simulink model "pendulum"  (R2020b)
settings: Solver=ode45  StartTime=0.0  StopTime=1000  FixedStep=0.01  RelTol=1e-3
InitFcn:
  | init_params
values from neighbouring files (symbols this model uses):
  b = 0.15    [init_params.m]
  g = 9.8    [init_params.m]
  I = 6250000    [init_params.m]
  L = 25    [init_params.m]
  m = 30000    [init_params.m]
  M = 20000    [init_params.m]
libraries: fuzblock x2, simulink_extras x2
settings Model: Creator=Administrator  LastModifiedBy=HZQ
settings SolverCC: ZeroCrossAlgorithm=Adaptive
settings DataIOCC: ReturnWorkspaceOutputs=off
settings DebuggingCC: ArithmeticOperatorsInVariantConditions=warning
settings SFSimCC: CustomCodeUndefinedFunction=UseInterfaceOnly

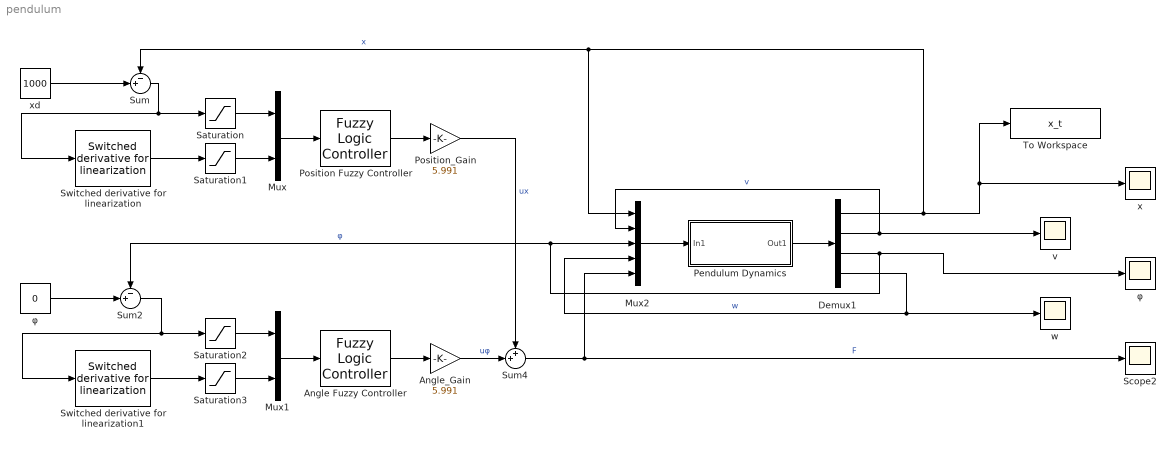
== system pendulum ==
  Angle Fuzzy Controller : fuzblock/Fuzzy Logic  Controller  FIS='angle_fuzzy_trimf.fis'  OutputSampleNumber=101  DataType=double  FuzzifiedInputs=off  RuleFiringStrengths=off  RuleOutputs=off  AggregatedOutputs=off  SimulateUsing=Interpreted execution  OutOfRangeInputValueMessage=warning  NoRuleFiredMessage=warning  EmptyOutputFuzzySetMessage=warning
  Angle_Gain : Gain  Gain=5.991
  Demux1 : Demux
  Mux : Mux  Inputs=2
  Mux1 : Mux  Inputs=2
  Mux2 : Mux  Inputs=5
  Pendulum Dynamics : Subsystem
  Position Fuzzy Controller : fuzblock/Fuzzy Logic  Controller  FIS='position_fuzzy_trimf.fis'  OutputSampleNumber=101  DataType=double  FuzzifiedInputs=off  RuleFiringStrengths=off  RuleOutputs=off  AggregatedOutputs=off  SimulateUsing=Interpreted execution  OutOfRangeInputValueMessage=warning  NoRuleFiredMessage=warning  EmptyOutputFuzzySetMessage=warning
  Position_Gain : Gain  Gain=5.991
  Saturation : Saturate  UpperLimit=1200  LowerLimit=-1200
  Saturation1 : Saturate  UpperLimit=10  LowerLimit=-10
  Saturation2 : Saturate  UpperLimit=6  LowerLimit=-6
  Saturation3 : Saturate  UpperLimit=6  LowerLimit=-6
  Scope2 : Scope
  Sum : Sum  Inputs=-+|
  Sum2 : Sum  Inputs=-+|
  Sum4 : Sum  Inputs=++|
  Switched derivative for linearization : simulink_extras/Linearization/Switched derivative for linearization  switchVal=0  derivConst=100
      settings: SourceProductBaseCode=SL
  Switched derivative for linearization1 : simulink_extras/Linearization/Switched derivative for linearization  switchVal=0  derivConst=100
      settings: SourceProductBaseCode=SL
  To Workspace : ToWorkspace  VariableName=x_t  SaveFormat=Timeseries  SampleTime=-1
  v : Scope
  w : Scope
  x : Scope
  "xd " : Constant  Value=1000  OutDataTypeStr=Inherit: Inherit via back propagation
  φ : Scope
  "φ " : Constant  Value=0  OutDataTypeStr=Inherit: Inherit via back propagation
  wires:
  Mux1/1 -> Angle Fuzzy Controller/1
  Mux/1 -> Position Fuzzy Controller/1
  Pendulum Dynamics/1(Out1) -> Demux1/1
  Demux1/1 -> x/1, To Workspace/1, Sum/1, Mux2/1  "x"
  "xd "/1 -> Sum/2
  Demux1/3 -> Sum2/1, Mux2/3, φ/1  "φ"
  "φ "/1 -> Sum2/2
  Mux2/1 -> Pendulum Dynamics/1(In1)
  Sum4/1 -> Mux2/5, Scope2/1  "F"
  Position Fuzzy Controller/1 -> Position_Gain/1
  Angle Fuzzy Controller/1 -> Angle_Gain/1
  Sum/1 -> Saturation/1, Switched derivative for linearization/1
  Sum2/1 -> Saturation2/1, Switched derivative for linearization1/1
  Position_Gain/1 -> Sum4/1  "ux"
  Angle_Gain/1 -> Sum4/2  "uφ"
  Demux1/2 -> v/1, Mux2/2  "v"
  Demux1/4 -> w/1, Mux2/4  "w"
  Switched derivative for linearization1/1 -> Saturation3/1
  Switched derivative for linearization/1 -> Saturation1/1
  Saturation/1 -> Mux/1
  Saturation1/1 -> Mux/2
  Saturation2/1 -> Mux1/1
  Saturation3/1 -> Mux1/2

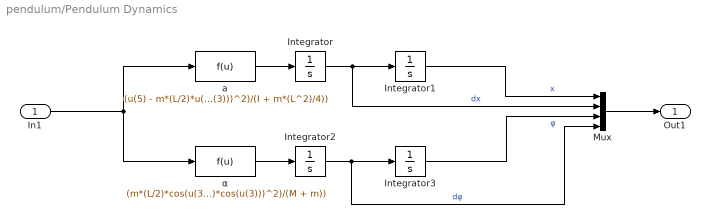
== system pendulum/Pendulum Dynamics ==
  In1 : Inport
  Integrator{,1..3} (4 alike) : Integrator
  Mux : Mux
  a : Fcn  Expr=(u(5) - m*(L/2)*u(4)^2*sin(u(3)) - b*u(2) - ((m*(L/2))^2*g*sin(u(3))*cos(u(3)))/(I + m*(L^2)/4)) / (M + m - ((m*(L/2)*cos(u(3)))^2)/(I + m*(L^2)/4))
  α : Fcn  Expr=(m*(L/2)*cos(u(3))*((u(5) - m*(L/2)*u(4)^2*sin(u(3)) - b*u(2))/(M + m)) - m*g*(L/2)*sin(u(3))) / (I + m*(L^2)/4 - ((m*(L/2)*cos(u(3)))^2)/(M + m))
  Out1 : Outport  VectorParamsAs1DForOutWhenUnconnected=off
  wires:
  Integrator/1 -> Mux/2, Integrator1/1  "dx"
  In1/1 -> α/1, a/1
  a/1 -> Integrator/1
  α/1 -> Integrator2/1
  Mux/1 -> Out1/1
  Integrator1/1 -> Mux/1  "x"
  Integrator3/1 -> Mux/3  "φ"
  Integrator2/1 -> Mux/4, Integrator3/1  "dφ"
